simulink model "trc_dyn"  (Simulink 10.3)
settings: Solver=ode45  StartTime=0.0  StopTime=8  MaxStep=0.1  RelTol=1e-3  AbsTol=1e-3
values from neighbouring files (symbols this model uses):
  a4 = 0.98    [vars_problem_17_to_21.m]    (also in vars_problem_18_to_21.m; vars_problem_8_to_16.m)
  d1 = 1.5    [vars_problem_17_to_21.m]    (also in vars_problem_18_to_21.m)
  n = 1    [vars_problem_17_to_21.m]    (also in vars_problem_18_to_21.m; vars_problem_8_to_16.m)
undefined symbols (not defined in the file): K_D, K_P
settings Model: Creator=Anders  LastModifiedBy=simon
settings SolverCC: AutoScaleAbsTol=off
settings DataIOCC: SaveOutput=off  TimeSaveName=t  SignalLoggingName=sigsOut
settings OptimizationCC: BooleanDataType=off  InitFltsAndDblsToZero=on
settings DebuggingCC: SaveWithParameterizedLinksMsg=none  MultiTaskDSMMsg=warning  MultiTaskCondExecSysMsg=none
settings HardwareCC: TargetUnknown=on
settings GRTTargetCC: TargetFcnLib=ansi_tfl_tmw.mat

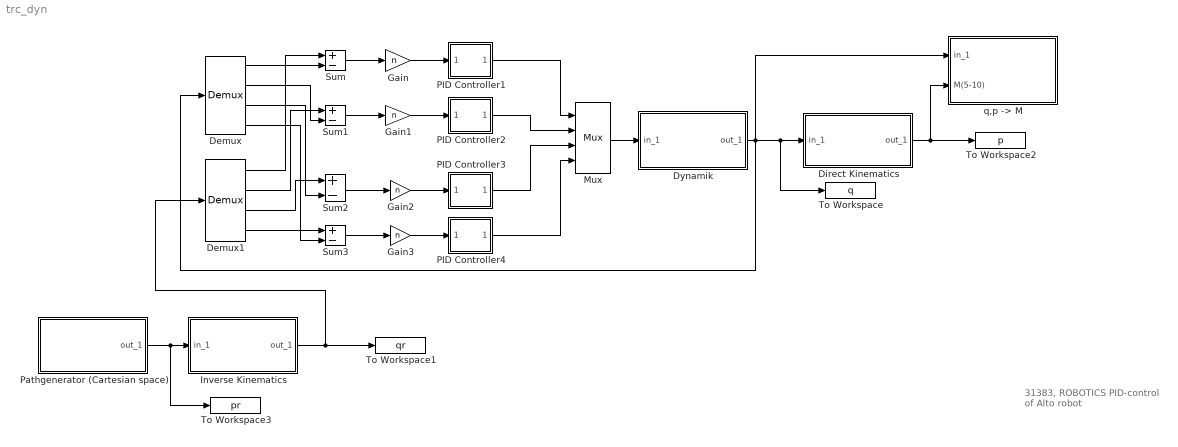
== system trc_dyn ==
  note: 31383, ROBOTICS
      |
      | PID-control of Alto robot
  Demux : Demux
      settings: DisplayOption=none
  Demux1 : Demux
      settings: DisplayOption=none
  Direct Kinematics : Subsystem
      mask Display: disp('Alto-Robot')
  Dynamik : Subsystem
      mask Display: disp('Alto-Robot\n tau -> q,q''')
  Gain{,1..3} (4 alike) : Gain  Gain=n  SaturateOnIntegerOverflow=on  OutDataTypeStr=Inherit: Same as input  ParamDataTypeStr=Inherit: Same as input
  Inverse Kinematics : Subsystem
      mask Display: disp('Alto-Robot')
  Mux : Mux
  PID Controller1 : Subsystem  mask(PID Controller){P=K_P(1), I=0, D=K_D(1)}
      mask prompts: P "Proportional:"; I "Integral"; D "Derivative:"
      mask help: Enter expressions for proportional, integral, and derivative terms.
      mask Help: This block implements a PID controller where parameters are entered for the Proportional, Integral and Derivative terms. Unmask this block to see how it works. The derivative term is implemented using a true derivative block.
      mask Display: disp('PID')
  PID Controller2 : Subsystem  mask(PID Controller){P=K_P(2), I=0, D=K_D(2)}
      mask prompts: P "Proportional:"; I "Integral"; D "Derivative:"
      mask help: Enter expressions for proportional, integral, and derivative terms.
      mask Help: This block implements a PID controller where parameters are entered for the Proportional, Integral and Derivative terms. Unmask this block to see how it works. The derivative term is implemented using a true derivative block.
      mask Display: disp('PID')
  PID Controller3 : Subsystem  mask(PID Controller){P=K_P(3), I=0, D=K_D(3)}
      mask prompts: P "Proportional:"; I "Integral"; D "Derivative:"
      mask help: Enter expressions for proportional, integral, and derivative terms.
      mask Help: This block implements a PID controller where parameters are entered for the Proportional, Integral and Derivative terms. Unmask this block to see how it works. The derivative term is implemented using a true derivative block.
      mask Display: disp('PID')
  PID Controller4 : Subsystem  mask(PID Controller){P=K_P(4), I=0, D=K_D(4)}
      mask prompts: P "Proportional:"; I "Integral"; D "Derivative:"
      mask help: Enter expressions for proportional, integral, and derivative terms.
      mask Help: This block implements a PID controller where parameters are entered for the Proportional, Integral and Derivative terms. Unmask this block to see how it works. The derivative term is implemented using a true derivative block.
      mask Display: disp('PID')
  "Pathgenerator (Cartesian space) " : Subsystem
      mask Display: disp('Alto-Robot\nBane -> p')
  Sum{,1..3} (4 alike) : Sum  Inputs=+-  InputSameDT=on  SaturateOnIntegerOverflow=on  OutDataTypeStr=Inherit: Same as first input
  To Workspace : ToWorkspace  VariableName=q
      settings: MaxDataPoints=100000
  To Workspace1 : ToWorkspace  VariableName=qr
      settings: MaxDataPoints=10000
  To Workspace2 : ToWorkspace  VariableName=p
      settings: MaxDataPoints=100000
  To Workspace3 : ToWorkspace  VariableName=pr
      settings: MaxDataPoints=10000
  "q,p -> M" : Subsystem
      mask Display: disp('Gem til vis4link')
  wires:
  Sum2/1 -> Gain2/1
  Sum1/1 -> Gain1/1
  PID Controller3/1(Out_1) -> Mux/3
  PID Controller2/1(Out_1) -> Mux/2
  Sum/1 -> Gain/1
  Mux/1 -> Dynamik/1(in_1)
  Inverse Kinematics/1(out_1) -> To Workspace1/1, Demux1/1
  Gain/1 -> PID Controller1/1(In_1)
  Gain1/1 -> PID Controller2/1(In_1)
  Gain2/1 -> PID Controller3/1(In_1)
  "Pathgenerator (Cartesian space) "/1(out_1) -> Inverse Kinematics/1(in_1), To Workspace3/1
  Direct Kinematics/1(out_1) -> "q,p -> M"/2(M(5-10)), To Workspace2/1
  Dynamik/1(out_1) -> Direct Kinematics/1(in_1), To Workspace/1, "q,p -> M"/1(in_1), Demux/1
  PID Controller1/1(Out_1) -> Mux/1
  Demux1/1 -> Sum/1
  Demux1/2 -> Sum1/1
  Demux1/3 -> Sum2/1
  Demux/1 -> Sum/2
  Demux/2 -> Sum1/2
  Demux/3 -> Sum2/2
  Sum3/1 -> Gain3/1
  Gain3/1 -> PID Controller4/1(In_1)
  PID Controller4/1(Out_1) -> Mux/4
  Demux1/4 -> Sum3/1
  Demux/4 -> Sum3/2

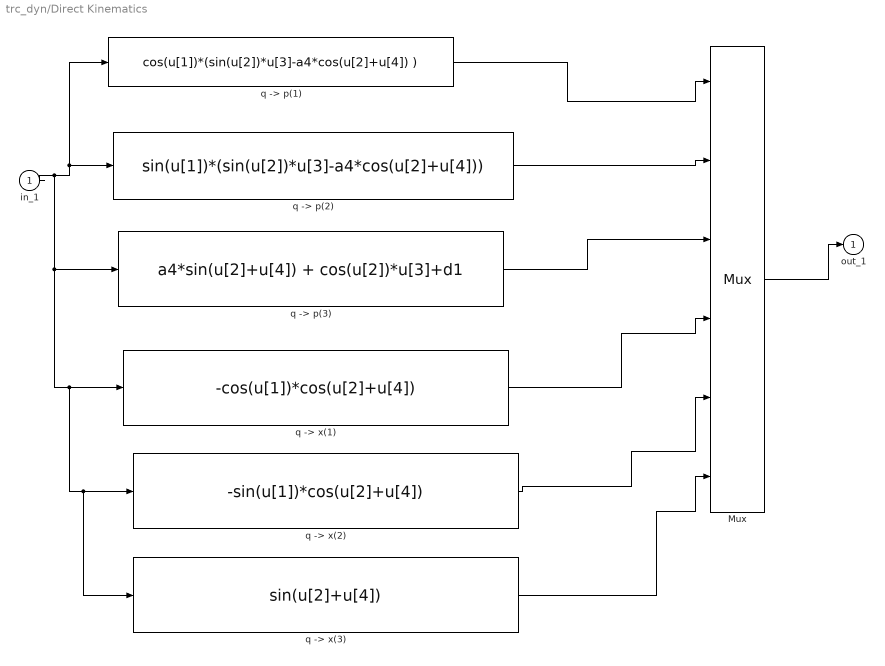
== system trc_dyn/Direct Kinematics ==
  in_1 : Inport
  Mux : Mux  Inputs=6
  "q -> p(1)" : Fcn  Expr=cos(u[1])*(sin(u[2])*u[3]-a4*cos(u[2]+u[4]) )
  "q -> p(2)" : Fcn  Expr=sin(u[1])*(sin(u[2])*u[3]-a4*cos(u[2]+u[4]))
  "q -> p(3)" : Fcn  Expr=a4*sin(u[2]+u[4]) + cos(u[2])*u[3]+d1
  "q -> x(1)" : Fcn  Expr=-cos(u[1])*cos(u[2]+u[4])
  "q -> x(2)" : Fcn  Expr=-sin(u[1])*cos(u[2]+u[4])
  "q -> x(3)" : Fcn  Expr=sin(u[2]+u[4])
  out_1 : Outport  InitialOutput=0  VectorParamsAs1DForOutWhenUnconnected=off
  wires:
  "q -> p(3)"/1 -> Mux/3
  "q -> p(2)"/1 -> Mux/2
  "q -> p(1)"/1 -> Mux/1
  "q -> x(1)"/1 -> Mux/4
  "q -> x(2)"/1 -> Mux/5
  "q -> x(3)"/1 -> Mux/6
  in_1/1 -> "q -> p(1)"/1, "q -> p(2)"/1, "q -> p(3)"/1, "q -> x(1)"/1, "q -> x(2)"/1, "q -> x(3)"/1
  Mux/1 -> out_1/1

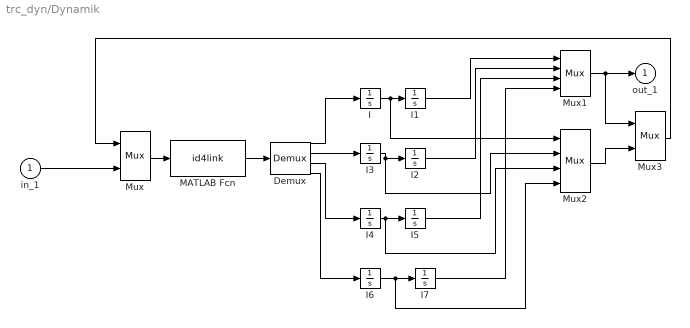
== system trc_dyn/Dynamik ==
  in_1 : Inport
  Demux : Demux
      settings: DisplayOption=none
  I{,1..7} (8 alike) : Integrator
  MATLAB Fcn : MATLABFcn  MATLABFcn=id4link  OutputDimensions=4
  Mux : Mux  Inputs=[8 4]
  Mux1 : Mux
  Mux2 : Mux
  Mux3 : Mux  Inputs=[4 4]
  out_1 : Outport  VectorParamsAs1DForOutWhenUnconnected=off
  wires:
  Mux1/1 -> out_1/1, Mux3/1
  Mux3/1 -> Mux/1
  I1/1 -> Mux1/1
  I5/1 -> Mux1/3
  I2/1 -> Mux1/2
  Demux/3 -> I4/1
  I4/1 -> Mux2/3, I5/1
  Demux/2 -> I3/1
  I3/1 -> Mux2/2, I2/1
  I/1 -> Mux2/1, I1/1
  Demux/1 -> I/1
  MATLAB Fcn/1 -> Demux/1
  Mux/1 -> MATLAB Fcn/1
  I6/1 -> I7/1, Mux2/4
  Demux/4 -> I6/1
  I7/1 -> Mux1/4
  Mux2/1 -> Mux3/2
  in_1/1 -> Mux/2

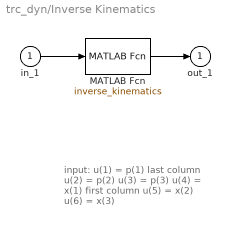
== system trc_dyn/Inverse Kinematics ==
  note: input:
      | u(1) = p(1) last column
      | u(2) = p(2)
      | u(3) = p(3)
      | u(4) = x(1) first column
      | u(5) = x(2)
      | u(6) = x(3)
  in_1 : Inport
  MATLAB Fcn : MATLABFcn  MATLABFcn=inverse_kinematics  OutputDimensions=4
  out_1 : Outport  VectorParamsAs1DForOutWhenUnconnected=off
  wires:
  MATLAB Fcn/1 -> out_1/1
  in_1/1 -> MATLAB Fcn/1

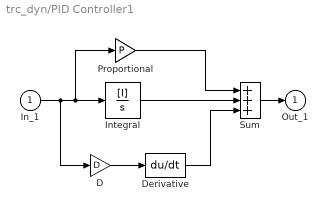
== system trc_dyn/PID Controller1 ==
  In_1 : Inport
  D : Gain  Gain=D  SaturateOnIntegerOverflow=on  OutDataTypeStr=Inherit: Same as input  ParamDataTypeStr=Inherit: Same as input
  Derivative : Derivative
  Integral : TransferFcn  Numerator=[I]  Denominator=[1 0]
  Proportional : Gain  Gain=P  SaturateOnIntegerOverflow=on  OutDataTypeStr=Inherit: Same as input  ParamDataTypeStr=Inherit: Same as input
  Sum : Sum  Inputs=+++  InputSameDT=on  SaturateOnIntegerOverflow=on  OutDataTypeStr=Inherit: Same as first input
  Out_1 : Outport  InitialOutput=0  VectorParamsAs1DForOutWhenUnconnected=off
  wires:
  Proportional/1 -> Sum/1
  Integral/1 -> Sum/2
  Derivative/1 -> Sum/3
  In_1/1 -> Integral/1, Proportional/1, D/1
  Sum/1 -> Out_1/1
  D/1 -> Derivative/1

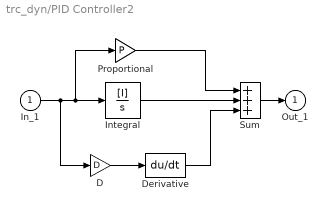
== system trc_dyn/PID Controller2 ==
  In_1 : Inport
  D : Gain  Gain=D  SaturateOnIntegerOverflow=on  OutDataTypeStr=Inherit: Same as input  ParamDataTypeStr=Inherit: Same as input
  Derivative : Derivative
  Integral : TransferFcn  Numerator=[I]  Denominator=[1 0]
  Proportional : Gain  Gain=P  SaturateOnIntegerOverflow=on  OutDataTypeStr=Inherit: Same as input  ParamDataTypeStr=Inherit: Same as input
  Sum : Sum  Inputs=+++  InputSameDT=on  SaturateOnIntegerOverflow=on  OutDataTypeStr=Inherit: Same as first input
  Out_1 : Outport  InitialOutput=0  VectorParamsAs1DForOutWhenUnconnected=off
  wires:
  Proportional/1 -> Sum/1
  Integral/1 -> Sum/2
  Derivative/1 -> Sum/3
  In_1/1 -> Integral/1, Proportional/1, D/1
  Sum/1 -> Out_1/1
  D/1 -> Derivative/1

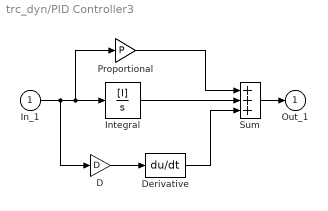
== system trc_dyn/PID Controller3 ==
  In_1 : Inport
  D : Gain  Gain=D  SaturateOnIntegerOverflow=on  OutDataTypeStr=Inherit: Same as input  ParamDataTypeStr=Inherit: Same as input
  Derivative : Derivative
  Integral : TransferFcn  Numerator=[I]  Denominator=[1 0]
  Proportional : Gain  Gain=P  SaturateOnIntegerOverflow=on  OutDataTypeStr=Inherit: Same as input  ParamDataTypeStr=Inherit: Same as input
  Sum : Sum  Inputs=+++  InputSameDT=on  SaturateOnIntegerOverflow=on  OutDataTypeStr=Inherit: Same as first input
  Out_1 : Outport  InitialOutput=0  VectorParamsAs1DForOutWhenUnconnected=off
  wires:
  D/1 -> Derivative/1
  Sum/1 -> Out_1/1
  In_1/1 -> D/1, Integral/1, Proportional/1
  Derivative/1 -> Sum/3
  Integral/1 -> Sum/2
  Proportional/1 -> Sum/1

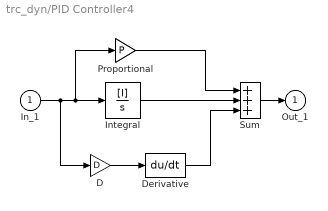
== system trc_dyn/PID Controller4 ==
  In_1 : Inport
  D : Gain  Gain=D  SaturateOnIntegerOverflow=on  OutDataTypeStr=Inherit: Same as input  ParamDataTypeStr=Inherit: Same as input
  Derivative : Derivative
  Integral : TransferFcn  Numerator=[I]  Denominator=[1 0]
  Proportional : Gain  Gain=P  SaturateOnIntegerOverflow=on  OutDataTypeStr=Inherit: Same as input  ParamDataTypeStr=Inherit: Same as input
  Sum : Sum  Inputs=+++  InputSameDT=on  SaturateOnIntegerOverflow=on  OutDataTypeStr=Inherit: Same as first input
  Out_1 : Outport  InitialOutput=0  VectorParamsAs1DForOutWhenUnconnected=off
  wires:
  Proportional/1 -> Sum/1
  Integral/1 -> Sum/2
  Derivative/1 -> Sum/3
  In_1/1 -> Proportional/1, Integral/1, D/1
  Sum/1 -> Out_1/1
  D/1 -> Derivative/1

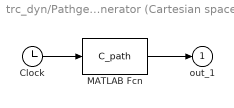
== system trc_dyn/Pathgenerator (Cartesian space)  ==
  Clock : Clock
  MATLAB Fcn : MATLABFcn  MATLABFcn=C_path  OutputDimensions=6
  out_1 : Outport  VectorParamsAs1DForOutWhenUnconnected=off
  wires:
  MATLAB Fcn/1 -> out_1/1
  Clock/1 -> MATLAB Fcn/1

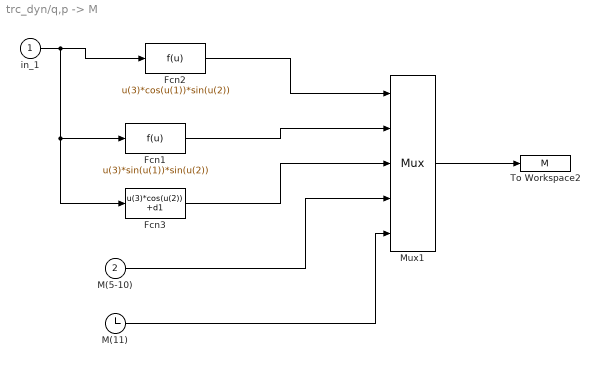
== system trc_dyn/q,p -> M ==
  in_1 : Inport
  M(5-10) : Inport  Port=2
  Fcn1 : Fcn  Expr=u(3)*sin(u(1))*sin(u(2))
  Fcn2 : Fcn  Expr=u(3)*cos(u(1))*sin(u(2))
  Fcn3 : Fcn  Expr=u(3)*cos(u(2)) +d1
  M(11) : Clock
  Mux1 : Mux  Inputs=[1 1 1 6 1]
  To Workspace2 : ToWorkspace  VariableName=M
      settings: MaxDataPoints=100000
  wires:
  Mux1/1 -> To Workspace2/1
  in_1/1 -> Fcn2/1, Fcn1/1, Fcn3/1
  Fcn2/1 -> Mux1/1
  Fcn1/1 -> Mux1/2
  Fcn3/1 -> Mux1/3
  M(5-10)/1 -> Mux1/4
  M(11)/1 -> Mux1/5
